simulink model "gucboost"  (R2022b)
settings: Solver=VariableStepAuto  StartTime=0.0  StopTime=0.1  RelTol=1e-3
libraries: spsCurrentMeasurementLib x4, spsVoltageMeasurementLib x4, spsParallelRLCBranchLib x3, spsDCVoltageSourceLib x1, spsDiodeLib x1, spsMeanLib x1, spsMosfetLib x1, sps_lib x1
settings Model: Creator=isild  LastModifiedBy=isild

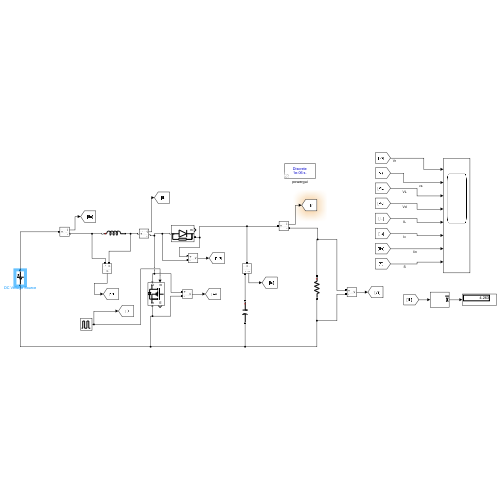
[thumbnail: Simulink's stored preview of the top-level diagram]
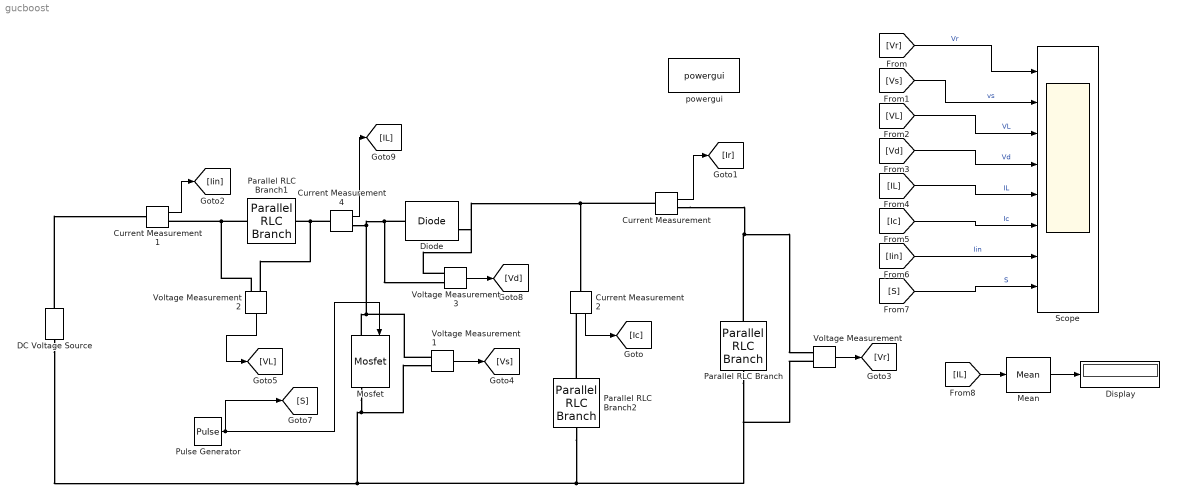
== system gucboost ==
  Current Measurement{,1..2,4} (4 alike) : spsCurrentMeasurementLib/Current Measurement  PhasorSimulation=off  OutputType=Complex  PSBequivalent=0
  DC Voltage Source : spsDCVoltageSourceLib/DC Voltage Source  Amplitude=25  Measurements=None
  Diode : spsDiodeLib/Diode  Ron=0.001  Lon=0  Vf=0.8  IC=0  UseSnubber=0  Rs=500  Cs=250e-9  Measurements=on
  Display : Display
  Mean : spsMeanLib/Mean  Freq=60  Vinit=0  Ts=0
  Mosfet : spsMosfetLib/Mosfet  Ron=0.1  Lon=0  Rd=0.01  Vfd=0  IC=0  Rs=1e5  Cs=inf  Measurements=on
  Parallel RLC Branch : spsParallelRLCBranchLib/Parallel RLC Branch  LConnTagsString=a  RConnTagsString=__new0  BranchType=R  Resistance=10  Inductance=1e-3  SetiL0=off  InitialCurrent=0  Capacitance=1e-6  Setx0=off  InitialVoltage=0  Measurements=None
  Parallel RLC Branch1 : spsParallelRLCBranchLib/Parallel RLC Branch  LConnTagsString=a  RConnTagsString=__new0  BranchType=L  Resistance=1  Inductance=0.047e-3  SetiL0=off  InitialCurrent=0  Capacitance=1e-6  Setx0=off  InitialVoltage=0  Measurements=None
  Parallel RLC Branch2 : spsParallelRLCBranchLib/Parallel RLC Branch  LConnTagsString=a  RConnTagsString=__new0  BranchType=C  Resistance=1  Inductance=1e-3  SetiL0=off  InitialCurrent=0  Capacitance=250e-6  Setx0=off  InitialVoltage=0  Measurements=None
  Pulse Generator : DiscretePulseGenerator  PulseType=Time based  Period=1/10000  PulseWidth=20
  Scope : Scope  NumInputPorts=8
  Voltage Measurement{,1..3} (4 alike) : spsVoltageMeasurementLib/Voltage Measurement  PhasorSimulation=off  OutputType=Complex  PSBequivalent=0
  powergui : sps_lib/powergui  Priority=1  SimulationMode=Discrete  SampleTime=1e-6  frequency=60  Iterations=50  frequencyindice=0  Pbase=100e6  ErrMax=1e-4  UnitsV=kV  UnitsW=MW  buscounter=0  FunctionMessages=off  echomessages=off  EnableUseOfTLC=off  CurrentSourceSwitches=off  DisableSnubberDevices=off  DisableRonSwitches=off  DisableVfSwitches=off  DisplayEquations=off  AutomaticDiscreteSolvers=off  SolverType=Tustin/Backward Euler (TBE)  Interpol=off  ExternalGateDelay=off  methode=off  Ts=100  x0status=blocks  SPID=on  SwTol=0  HookPort=off  NonlinearTolerance=1e-4  nMaxIteration=100  ContinueOnMaxIteration=off  RestoreLinks=warning  ResistiveCurrentMeasurement=off  Frange=[0:2:500]  Ylog=off  Xlog=on  ShowGrid=off  save=off  variable=ZData  structure=0  ZoomFFT=off  StartTime=0.0  cycles=1  DisplayStyle=1  fundamental=60  FreqAxis=off  MaxFrequency=1000  frequencyindicesteady=1  RmsSteady=1  display=off
  wires:
  Current Measurement/1 -> [Ir]
  Current Measurement2/1 -> [Ic]
  Voltage Measurement3/1 -> [Vd]
  Current Measurement1/1 -> [Iin]
  Pulse Generator/1 -> Mosfet/1, [S]
  Voltage Measurement2/1 -> [VL]
  Voltage Measurement1/1 -> [Vs]
  Voltage Measurement/1 -> [Vr]
  Current Measurement4/1 -> [IL]
  [Vs] -> Scope/2  "vs"
  [VL] -> Scope/3  "VL"
  [Vd] -> Scope/4  "Vd"
  [IL] -> Scope/5  "IL"
  [Ic] -> Scope/6  "Ic"
  [Iin] -> Scope/7  "Iin"
  [S] -> Scope/8  "S"
  [IL] -> Mean/1
  Mean/1 -> Display/1
  [Vr] -> Scope/1  "Vr"
  connections:
  Voltage Measurement1/LConn1 -- Mosfet/LConn1 -- Current Measurement4/RConn1 -- Diode/LConn1 -- Voltage Measurement3/LConn2
  Current Measurement/RConn1 -- Parallel RLC Branch/LConn1 -- Voltage Measurement/LConn1
  Parallel RLC Branch2/RConn1 -- DC Voltage Source/LConn1 -- Mosfet/RConn1 -- Voltage Measurement1/LConn2 -- Voltage Measurement/LConn2 -- Parallel RLC Branch/RConn1
  Current Measurement/LConn1 -- Voltage Measurement3/LConn1 -- Diode/RConn1 -- Current Measurement2/LConn1
  Voltage Measurement2/LConn2 -- Parallel RLC Branch1/LConn1 -- Current Measurement1/RConn1
  DC Voltage Source/RConn1 -- Current Measurement1/LConn1
  Parallel RLC Branch2/LConn1 -- Current Measurement2/RConn1
  Voltage Measurement2/LConn1 -- Current Measurement4/LConn1 -- Parallel RLC Branch1/RConn1
